simulink model "simulation"  (R2017a)
settings: Solver=VariableStepAuto  StartTime=0.0  StopTime=50  RelTol=1e-3
libraries: simulink x1
settings Model: Creator=Moustafa7  LastModifiedBy=Moustafa7

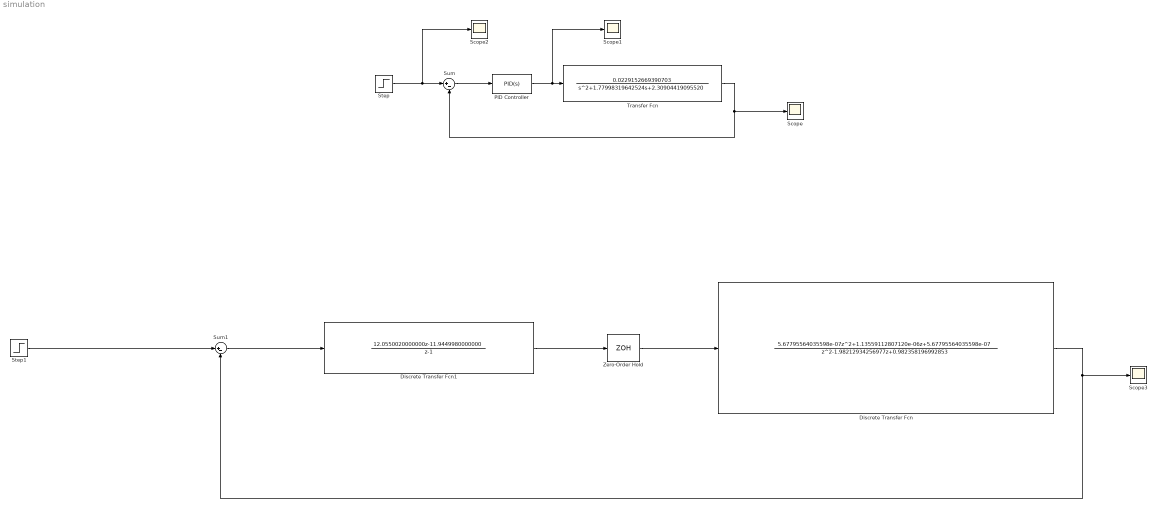
== system simulation ==
  Discrete Transfer Fcn : DiscreteTransferFcn  Numerator=[5.67795564035598e-07,1.13559112807120e-06,5.67795564035598e-07]  Denominator=[1,-1.98212934256977,0.982358196992853]
  Discrete Transfer Fcn1 : DiscreteTransferFcn  Numerator=[12.0550020000000,-11.9449980000000]  Denominator=[1,-1]
  PID Controller : simulink/Continuous/PID Controller  Controller=PID  TimeDomain=Continuous-time  SampleTime=-1  IntegratorMethod=Forward Euler  FilterMethod=Forward Euler  Form=Parallel  UseFilter=on  ControllerParametersSource=internal  P=12  I=11  D=0  N=100  InitialConditionSource=internal  InitialConditionForIntegrator=0  InitialConditionForFilter=0  ExternalReset=none  LimitOutput=off  UpperSaturationLimit=inf  LowerSaturationLimit=-inf  LinearizeAsGain=on  AntiWindupMode=none  Kb=1  TrackingMode=off  Kt=1  PParamMin=[]  PParamMax=[]  IParamMin=[]  IParamMax=[]  DParamMin=[]  DParamMax=[]  NParamMin=[]  NParamMax=[]  KbParamMin=[]  KbParamMax=[]  KtParamMin=[]  KtParamMax=[]  POutMin=[]  POutMax=[]  IOutMin=[]  IOutMax=[]  DOutMin=[]  DOutMax=[]  NOutMin=[]  NOutMax=[]  KbOutMin=[]  KbOutMax=[]  KtOutMin=[]  KtOutMax=[]  IntegratorOutMin=[]  IntegratorOutMax=[]  FilterOutMin=[]  FilterOutMax=[]  SumOutMin=[]  SumOutMax=[]  SumI1OutMin=[]  SumI1OutMax=[]  SumI2OutMin=[]  SumI2OutMax=[]  SumI3OutMin=[]  SumI3OutMax=[]  SumDOutMin=[]  SumDOutMax=[]  SaturationOutMin=[]  SaturationOutMax=[]  IntegratorContinuousStateAttributes=''  IntegratorStateMustResolveToSignalObject=off  IntegratorRTWStateStorageClass=Auto  FilterContinuousStateAttributes=''  FilterStateMustResolveToSignalObject=off  FilterRTWStateStorageClass=Auto  DifferentiatorICPrevScaledInput=0  DifferentiatorOutMin=[]  DifferentiatorOutMax=[]  InitialConditionSetting=State (most efficient)
  Scope{,1..3} (4 alike) : Scope
  Step : Step  After=15  SampleTime=0
  Step1 : Step  After=15  SampleTime=0
  Sum : Sum  Inputs=|+-
  Sum1 : Sum  Inputs=|+-
  Transfer Fcn : TransferFcn  Numerator=[0,0,0.0229152669390703]  Denominator=[1,1.77998319642524,2.30904419095520]
  Zero-Order Hold : ZeroOrderHold  SampleTime=0.01
  wires:
  Sum/1 -> PID Controller/1
  Step/1 -> Scope2/1, Sum/1
  PID Controller/1 -> Scope1/1, Transfer Fcn/1
  Transfer Fcn/1 -> Sum/2, Scope/1
  Zero-Order Hold/1 -> Discrete Transfer Fcn/1
  Discrete Transfer Fcn1/1 -> Zero-Order Hold/1
  Discrete Transfer Fcn/1 -> Sum1/2, Scope3/1
  Step1/1 -> Sum1/1
  Sum1/1 -> Discrete Transfer Fcn1/1
